simulink model "DYC_controller"  (R2018b)
settings: Solver=FixedStepAuto  StartTime=0.0  StopTime=inf  FixedStep=Ts  RelTol=1e-3  EnableMultiTasking=on
values from neighbouring files (symbols this model uses):
  A_vte = [1 0 -2*Ts*m_s/WB*(l_r*h_rc_f/w1+l_f*h_rc_r/w2) 0 -2*Ts*(K_f/w1+K_r/w2) ... (first row only)    [main.m]
  A_vte_p2 = [1 0 0 0 0 -Ts * m * hc / 2 / WB 0 -Ts * l_r * m * hc / WB / w1 ... (first row only)    [main.m]
  b1 = ones(4,1)/R    [main.m]
  boundary = 3000    [main.m]
  C_vte = [0 1 0 g 0 ... (first row only)    [main.m]
  C_vte_p2 = [1, -1, 1, -1, 0, 0, 0, 0 ... (first row only)    [main.m]
  eta = 0    [main.m]
  F_z1_s = l_r * m * g / 2 / WB    (= 9.45353456158)    [main.m]
  F_z2_s = F_z1_s    (= 9.45353456158)    [main.m]
  F_z3_s = l_f * m * g / 2 / WB    (= 9.11094809852)    [main.m]
  F_z4_s = F_z3_s    (= 9.11094809852)    [main.m]
  g = 9.81    [main.m]
  h_rc_f = 0.00    (= 0)    [main.m]
  h_rc_r = 0.00    (= 0)    [main.m]
  hc = 0.0751    [main.m]
  J = 0.9    [main.m]
  k1 = 2000    [main.m]
  k2 = 1000    [main.m]
  K_f = K_lin*l_cs^2*cos(phi*pi/180)    [main.m]
  K_r = K_lin*l_cs^2*cos(phi*pi/180)    [main.m]
  Kd = 0    [main.m]
  Ki = 75    [main.m]
  Kp = 600    [main.m]
  l_f = 0.1968    [main.m]
  l_r = 0.2042    [main.m]
  m = 3.832    [main.m]
  m_s = 0.9*m    (= 3.4488)    [main.m]
  mu = 0.8    [main.m]
  Protean_PD18_motormap = [2.92104016907 601.978033502 650.789692516 685.109940533 725.756581133 754.659963437 780.850883334 807.9513301 837.761936672 868.484372712 893.788791739 922.70944354 ... (50 elements, 25x2)]    [Protean_PD18_motormap.mat]
  Q_lat_process = 1E0*[var_r^2  0 0 0 0 0 0 0 0 ... (first row only)    [main.m]
  Q_lat_sensor = 1E-2*[var_r_s^2 0 0 0 ... (first row only)    [main.m]
  Q_meas_susp_p1 = [var_ay_m_p^2 0 0 0 ... (first row only)    [main.m]
  Q_meas_susp_p2 = [var_del_Fz^2 0 0 0 0 ... (first row only)    [main.m]
  R = 0.055    [main.m]
  Ts = 0.015    [main.m]
  V_x0 = (1000/3600)*V_x0    (= 11.1111111111)    [main.m]
  w1 = 0.2824    [main.m]
  w2 = 2.929    [main.m]
  WB = 0.406    [main.m]
undefined symbols (not defined in the file or in its folder): C_lf, C_lr, DiscIntNeverNeededParam, Discrete, t_e, Time
libraries: raspberrypilib x24, hdlsllib x21, simulink x17, discretizing x2, ctrlSharedLib x2, sharedTrackingLibrary x1
(part 3 of 3)

== system DYC_controller/Hardware/SSIV Hardware Communication/gyr_z read message (Master --> Slave) ==
  Inport : Inport
  Mux : Mux
      settings: DisplayOption=signals
  Read Bit Set : simulink/Logic and Bit Operations/Bit Set  iBit=7
      settings: SourceProductName=Simulink  SourceProductBaseCode=SL
  uint8_t 1 : Constant  OutDataTypeStr=uint8
  uint8_t 2 : Constant  OutDataTypeStr=uint8
  uint8_t 3 : Constant  OutDataTypeStr=uint8
  Out1 : Outport
  wires:
  uint8_t 2/1 -> Mux/3  "Byte 0 will be returned here"
  Mux/1 -> Out1/1
  uint8_t 3/1 -> Mux/4  "Byte 1 will be returned here"
  Inport/1 -> Read Bit Set/1
  uint8_t 1/1 -> Mux/2  "Junk will be returned here"
  Read Bit Set/1 -> Mux/1  "Addres/RW Byte gyr_z Teensy Status will be returned here"

== system DYC_controller/Hardware/SSIV Hardware Communication/gyr_z return message (Slave --> Master) ==
  In1 : Inport
  8 bytes concatinated converted to double : DataTypeConversion  OutDataTypeStr=double
  Bit Concat : hdlsllib/Logic and Bit Operations/Bit Concat  numInputs=2
      settings: SourceProductName=HDL Coder  SourceProductBaseCode=HD
  Bytes of the return message : Display
      settings: Format=decimal (Stored Integer)
  Data Type Conversion : DataTypeConversion  OutDataTypeStr=int16  RndMeth=Nearest
  Demux : Demux
  Display : Display
      settings: Format=binary (Stored Integer)
  Display1 : Display
      settings: Format=decimal (Stored Integer)
  Display2 : Display
      settings: Format=binary (Stored Integer)
  Gyroscope Int to Double Scale Factor : Gain  Gain=1/900
  gyr_z : Outport
  wires:
  Gyroscope Int to Double Scale Factor/1 -> gyr_z/1, Display1/1
  Demux/3 -> Bit Concat/2
  Demux/4 -> Bit Concat/1
  Bit Concat/1 -> Data Type Conversion/1
  In1/1 -> Demux/1, Bytes of the return message/1
  Demux/1 -> Display/1  "Previous Data"
  Demux/2 -> Display2/1  "Slave Status"
  8 bytes concatinated converted to double/1 -> Gyroscope Int to Double Scale Factor/1  "gyr_z"
  Data Type Conversion/1 -> 8 bytes concatinated converted to double/1

== system DYC_controller/Hardware/SSIV Hardware Communication/radio_steering read message (Master --> Slave) ==
  Inport : Inport
  Mux : Mux
      settings: DisplayOption=signals
  Read Bit Set : simulink/Logic and Bit Operations/Bit Set  iBit=7
      settings: SourceProductName=Simulink  SourceProductBaseCode=SL
  uint8_t 1 : Constant  OutDataTypeStr=uint8
  uint8_t 2 : Constant  OutDataTypeStr=uint8
  uint8_t 3 : Constant  OutDataTypeStr=uint8
  Out1 : Outport
  wires:
  Read Bit Set/1 -> Mux/1  "Addres/RW Byte radio_steering Teensy Status will be returned here"
  uint8_t 1/1 -> Mux/2  "Junk will be returned here"
  Inport/1 -> Read Bit Set/1
  uint8_t 3/1 -> Mux/4  "Byte 1 will be returned here"
  Mux/1 -> Out1/1
  uint8_t 2/1 -> Mux/3  "Byte 0 will be returned here"

== system DYC_controller/Hardware/SSIV Hardware Communication/radio_steering return message (Slave --> Master) ==
  In1 : Inport
  8 bytes concatinated converted to double : DataTypeConversion  OutDataTypeStr=double  RndMeth=Nearest
  Bit Concat : hdlsllib/Logic and Bit Operations/Bit Concat  numInputs=2
      settings: SourceProductName=HDL Coder  SourceProductBaseCode=HD
  Bytes of the return message : Display
      settings: Format=decimal (Stored Integer)
  Data Type Conversion : DataTypeConversion  OutDataTypeStr=int16  RndMeth=Nearest
  Demux : Demux
  Display : Display
      settings: Format=binary (Stored Integer)
  Display1 : Display
      settings: Format=decimal (Stored Integer)
  Display2 : Display
      settings: Format=binary (Stored Integer)
  radio_steering : Outport
  wires:
  8 bytes concatinated converted to double/1 -> Display1/1, radio_steering/1  "radio_steering"
  Demux/2 -> Display2/1  "Slave Status"
  Demux/1 -> Display/1  "Previous Data"
  In1/1 -> Bytes of the return message/1, Demux/1
  Bit Concat/1 -> Data Type Conversion/1
  Demux/4 -> Bit Concat/1
  Demux/3 -> Bit Concat/2
  Data Type Conversion/1 -> 8 bytes concatinated converted to double/1

== system DYC_controller/Hardware/SSIV Hardware Communication/radio_throttle read message (Master --> Slave) ==
  Inport : Inport
  Mux : Mux
      settings: DisplayOption=signals
  Read Bit Set : simulink/Logic and Bit Operations/Bit Set  iBit=7
      settings: SourceProductName=Simulink  SourceProductBaseCode=SL
  uint8_t 1 : Constant  OutDataTypeStr=uint8
  uint8_t 2 : Constant  OutDataTypeStr=uint8
  uint8_t 3 : Constant  OutDataTypeStr=uint8
  Out1 : Outport
  wires:
  Read Bit Set/1 -> Mux/1  "Address/RW Byte radio_throttle Teensy Status will be returned here"
  uint8_t 1/1 -> Mux/2  "Junk will be returned here"
  Inport/1 -> Read Bit Set/1
  uint8_t 3/1 -> Mux/4  "Byte 1 will be returned here"
  Mux/1 -> Out1/1
  uint8_t 2/1 -> Mux/3  "Byte 0 will be returned here"

== system DYC_controller/Hardware/SSIV Hardware Communication/radio_throttle return message (Slave --> Master) ==
  In1 : Inport
  8 bytes concatinated converted to double : DataTypeConversion  OutDataTypeStr=double  RndMeth=Nearest
  Bit Concat : hdlsllib/Logic and Bit Operations/Bit Concat  numInputs=2
      settings: SourceProductName=HDL Coder  SourceProductBaseCode=HD
  Bytes of the return message : Display
      settings: Format=decimal (Stored Integer)
  Data Type Conversion : DataTypeConversion  OutDataTypeStr=int16  RndMeth=Nearest
  Demux : Demux
  Display : Display
      settings: Format=binary (Stored Integer)
  Display1 : Display
      settings: Format=decimal (Stored Integer)
  Display2 : Display
      settings: Format=binary (Stored Integer)
  radio_throttle : Outport
  wires:
  8 bytes concatinated converted to double/1 -> Display1/1, radio_throttle/1  "radio_throttle"
  Demux/2 -> Display2/1  "Slave Status"
  Demux/1 -> Display/1  "Previous Data"
  In1/1 -> Bytes of the return message/1, Demux/1
  Bit Concat/1 -> Data Type Conversion/1
  Demux/4 -> Bit Concat/1
  Demux/3 -> Bit Concat/2
  Data Type Conversion/1 -> 8 bytes concatinated converted to double/1

== system DYC_controller/Hardware/SSIV Hardware Communication/servo_out Write Message (Master --> Slave) ==
  In1 : Inport
  Bit Slice2 : hdlsllib/Logic and Bit Operations/Bit Slice  lidx=15  ridx=8
  Bit Slice3 : hdlsllib/Logic and Bit Operations/Bit Slice  lidx=7  ridx=0
  Display5 : Display
      settings: Format=decimal (Stored Integer)
  Mux : Mux  Inputs=2
      settings: DisplayOption=signals
  Out1 : Outport
  wires:
  In1/1 -> Display5/1, Bit Slice3/1, Bit Slice2/1  "Servo"
  Mux/1 -> Out1/1
  Bit Slice3/1 -> Mux/1
  Bit Slice2/1 -> Mux/2

== system DYC_controller/Hardware/SSIV Hardware Communication/throttle_left_front Write Message (Master --> Slave) ==
  In1 : Inport
  Bit Slice : hdlsllib/Logic and Bit Operations/Bit Slice  lidx=15  ridx=8
  Bit Slice1 : hdlsllib/Logic and Bit Operations/Bit Slice  lidx=7  ridx=0
  Display4 : Display
  Mux : Mux  Inputs=2
      settings: DisplayOption=signals
  Output : Outport
  wires:
  Mux/1 -> Output/1
  Bit Slice/1 -> Display4/1, Mux/2
  Bit Slice1/1 -> Mux/1
  In1/1 -> Bit Slice/1, Bit Slice1/1

== system DYC_controller/Hardware/SSIV Hardware Communication/throttle_left_rear Write Message (Master --> Slave) ==
  In1 : Inport
  Bit Slice : hdlsllib/Logic and Bit Operations/Bit Slice  lidx=15  ridx=8
  Bit Slice1 : hdlsllib/Logic and Bit Operations/Bit Slice  lidx=7  ridx=0
  Display4 : Display
  Mux : Mux  Inputs=2
      settings: DisplayOption=signals
  Output : Outport
  wires:
  In1/1 -> Bit Slice1/1, Bit Slice/1
  Bit Slice1/1 -> Mux/1
  Bit Slice/1 -> Mux/2, Display4/1
  Mux/1 -> Output/1

== system DYC_controller/Hardware/SSIV Hardware Communication/throttle_right_front Write Message (Master --> Slave) ==
  In1 : Inport
  Bit Slice : hdlsllib/Logic and Bit Operations/Bit Slice  lidx=15  ridx=8
  Bit Slice1 : hdlsllib/Logic and Bit Operations/Bit Slice  lidx=7  ridx=0
  Display4 : Display
  Mux : Mux  Inputs=2
      settings: DisplayOption=signals
  Output : Outport
  wires:
  Mux/1 -> Output/1
  Bit Slice/1 -> Display4/1, Mux/2
  Bit Slice1/1 -> Mux/1
  In1/1 -> Bit Slice/1, Bit Slice1/1

== system DYC_controller/Hardware/SSIV Hardware Communication/throttle_right_rear Write Message (Master --> Slave) ==
  In1 : Inport
  Bit Slice : hdlsllib/Logic and Bit Operations/Bit Slice  lidx=15  ridx=8
  Bit Slice1 : hdlsllib/Logic and Bit Operations/Bit Slice  lidx=7  ridx=0
  Display4 : Display
  Mux : Mux  Inputs=2
      settings: DisplayOption=signals
  Output : Outport
  wires:
  In1/1 -> Bit Slice1/1, Bit Slice/1
  Bit Slice1/1 -> Mux/1
  Bit Slice/1 -> Mux/2, Display4/1
  Mux/1 -> Output/1

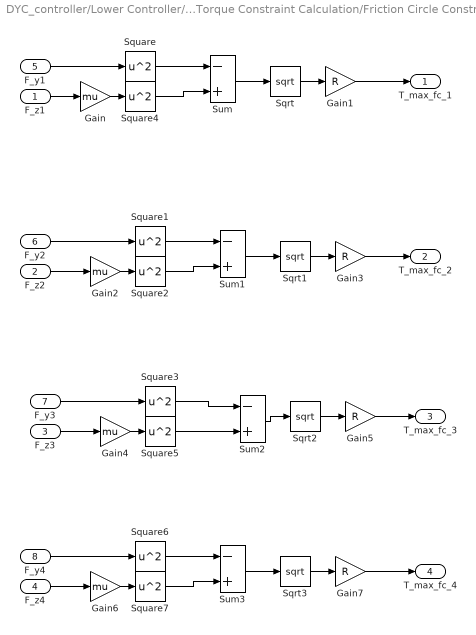
== system DYC_controller/Lower Controller/Torque Constraint Calculation/Friction Circle Constraint ==
  F_z1 : Inport
  F_z2 : Inport  Port=2
  F_z3 : Inport  Port=3
  F_z4 : Inport  Port=4
  F_y1 : Inport  Port=5
  F_y2 : Inport  Port=6
  F_y3 : Inport  Port=7
  F_y4 : Inport  Port=8
  Gain{,2,4,6} (4 alike) : Gain  Gain=mu
  Gain{1,3,5,7} (4 alike) : Gain  Gain=R
  Sqrt{,1..3} (4 alike) : Sqrt  SaturateOnIntegerOverflow=on
  Square{,1..7} (8 alike) : Math  Operator=square  SaturateOnIntegerOverflow=on
  Sum{,1..3} (4 alike) : Sum  Inputs=-+
  T_max_fc_1 : Outport
  T_max_fc_2 : Outport  Port=2
  T_max_fc_3 : Outport  Port=3
  T_max_fc_4 : Outport  Port=4
  wires:
  F_z1/1 -> Gain/1
  Gain3/1 -> T_max_fc_2/1
  F_y1/1 -> Square/1
  Gain/1 -> Square4/1
  Square/1 -> Sum/1
  Square4/1 -> Sum/2
  Sum/1 -> Sqrt/1
  Sqrt/1 -> Gain1/1
  Gain1/1 -> T_max_fc_1/1
  Sqrt1/1 -> Gain3/1
  Sum1/1 -> Sqrt1/1
  Square1/1 -> Sum1/1
  Gain2/1 -> Square2/1
  F_y2/1 -> Square1/1
  F_z2/1 -> Gain2/1
  Square2/1 -> Sum1/2
  Square5/1 -> Sum2/2
  F_z3/1 -> Gain4/1
  F_y3/1 -> Square3/1
  Gain4/1 -> Square5/1
  Square3/1 -> Sum2/1
  Sum2/1 -> Sqrt2/1
  Sqrt2/1 -> Gain5/1
  Gain5/1 -> T_max_fc_3/1
  Gain7/1 -> T_max_fc_4/1
  Sqrt3/1 -> Gain7/1
  Sum3/1 -> Sqrt3/1
  Square6/1 -> Sum3/1
  Gain6/1 -> Square7/1
  F_y4/1 -> Square6/1
  F_z4/1 -> Gain6/1
  Square7/1 -> Sum3/2

== system DYC_controller/Lower Controller/Torque Constraint Calculation/Motor Output Constraint ==
  omega_1 : Inport
  omega_2 : Inport  Port=2
  omega_3 : Inport  Port=3
  omega_4 : Inport  Port=4
  Gain{3..4,11..12} (4 alike) : Gain  Gain=60/(2*pi)
  PD18 Peak Torque : Lookup_n-D  NumberOfTableDimensions=1  BreakpointsForDimension1=Protean_PD18_motormap(:,1)  BreakpointsForDimension3=[5, 7]  Table=Protean_PD18_motormap(:,2)  InternalRulePriority=Speed  RndMeth=Simplest  InputSameDT=on
  n-D Lookup Table1 : Lookup_n-D  NumberOfTableDimensions=1  BreakpointsForDimension1=Protean_PD18_motormap(:,1)  BreakpointsForDimension3=[5, 7]  Table=Protean_PD18_motormap(:,2)  InternalRulePriority=Speed  RndMeth=Simplest  InputSameDT=on
  n-D Lookup Table2 : Lookup_n-D  NumberOfTableDimensions=1  BreakpointsForDimension1=Protean_PD18_motormap(:,1)  BreakpointsForDimension3=[5, 7]  Table=Protean_PD18_motormap(:,2)  InternalRulePriority=Speed  RndMeth=Simplest  InputSameDT=on
  n-D Lookup Table3 : Lookup_n-D  NumberOfTableDimensions=1  BreakpointsForDimension1=Protean_PD18_motormap(:,1)  BreakpointsForDimension3=[5, 7]  Table=Protean_PD18_motormap(:,2)  InternalRulePriority=Speed  RndMeth=Simplest  InputSameDT=on
  T_peak_motor_1 : Outport
  T_peak_motor_2 : Outport  Port=2
  T_peak_motor_3 : Outport  Port=3
  T_peak_motor_4 : Outport  Port=4
  wires:
  Gain3/1 -> PD18 Peak Torque/1
  omega_2/1 -> Gain4/1
  omega_1/1 -> Gain3/1
  Gain4/1 -> n-D Lookup Table1/1
  omega_4/1 -> Gain12/1
  Gain11/1 -> n-D Lookup Table2/1
  Gain12/1 -> n-D Lookup Table3/1
  omega_3/1 -> Gain11/1
  PD18 Peak Torque/1 -> T_peak_motor_1/1
  n-D Lookup Table1/1 -> T_peak_motor_2/1
  n-D Lookup Table2/1 -> T_peak_motor_3/1
  n-D Lookup Table3/1 -> T_peak_motor_4/1

== system DYC_controller/Lower Controller/Torque Constraint Calculation/Road Adhesion Constraint ==
  F_z1 : Inport
  F_z2 : Inport  Port=2
  F_z3 : Inport  Port=3
  F_z4 : Inport  Port=4
  Constant2 : Constant  Value=mu
  Gain6 : Gain  Gain=R
  Multiply{,1..3} (4 alike) : Product
  T_max_ad_1 : Outport
  T_max_ad_2 : Outport  Port=2
  T_max_ad_3 : Outport  Port=3
  T_max_ad_4 : Outport  Port=4
  wires:
  F_z1/1 -> Multiply/2
  F_z2/1 -> Multiply1/2
  F_z3/1 -> Multiply2/2
  Constant2/1 -> Gain6/1
  F_z4/1 -> Multiply3/2
  Gain6/1 -> Multiply/1, Multiply3/1, Multiply2/1, Multiply1/1
  Multiply/1 -> T_max_ad_1/1
  Multiply1/1 -> T_max_ad_2/1
  Multiply2/1 -> T_max_ad_3/1
  Multiply3/1 -> T_max_ad_4/1

== matlab function DYC_controller/Lower Controller/MATLAB Function ==
  settings: updateMethod=DISCRETE
  data: T_max input size=4; torque output size=4; M_des input; T_base input; V_wx input; b1 input; b2 input; C_lf input; C_lr input; R input; fval output; iter output; c_residual output; F_y input; F_z input
function [torque, fval, iter, c_residual] = Torque_Allocation(T_max, M_des, T_base, V_wx, b1, b2, C_lf, C_lr, R, F_y, F_z)
% This function solves a constrained optimization problem for optimal
% torque allocation which satisfies the yaw moment control signal
% Cost function: longitudinal slip power loss
% Method: Lagrangian algorithm
% Reference: Wei-Ta Chu, "Algorithms for Constrained Optimization"

V_wx_1 = V_wx(1);
V_wx_2 = V_wx(2);
V_wx_3 = V_wx(3);
V_wx_4 = V_wx(4);

C_l1 = C_lf;
C_l2 = C_lf;
C_l3 = C_lr;
C_l4 = C_lr;

T_min = - T_max;
x      = [0 0 0 0]';    % Initial guess for torque values

% Concatenate torque vectoring model vectors
B_TV = [ b1, b2 ]';
A    = B_TV;                    % Coefficient matrix
c    = [ T_base / R, M_des ]';       % Vector of control objectives
D    = [ V_wx_1 / (R ^ 2 * C_l1), 0, 0, 0;  % Slip power loss matrix
         0, V_wx_2 / (R ^ 2 * C_l2), 0, 0;
         0, 0, V_wx_3 / (R ^ 2 * C_l3), 0;
         0, 0, 0, V_wx_4 / (R ^ 2 * C_l4) ];

% T    = @(x) [x(1) x(2) x(3) x(4)]';
% Y    = @(F_y) [F_y(1) F_y(2) F_y(3) F_y(4)]';
% Z    = @(F_z) [1/F_z(1) 1/F_z(2) 1/F_z(3) 1/F_z(4)];
% X    = @(x) [x(1) 0 0 0;
%              0 x(2) 0 0;
%              0 0 x(3) 0;
%              0 0 0 x(4)];
% W    = @(F_y) [F_y(1) 0 0 0;
%                0 F_y(2) 0 0;
%                0 0 F_y(3) 0;
%                0 0 0 F_y(4)];
%      
  
% Objective function F(x) to minimize
% Slip power loss
F  = @(x) x' * D * x;
dF = @(x) 2 * D * x;

% % Vertical load matching
% F = @(x, F_z) 0.5*x'*Q*x + (x(1)/(x(1)+x(3)) - (F_z(1)/(F_z(1) + F_z(3))))^2 + (x(2)/(x(2)+x(4))...
%     -F_z(2)/(F_z(2)+F_z(4)))^2;
% 
% dF = @(x, F_z) [-2*(x(1)/(x(1) + x(3)) - F_z(1)/(F_z(1) + F_z(3)))*(x(1)/(x(1) + x(3))^2 -...
%                 1/(x(1) + x(3)));
%                 -2*(x(2)/(x(2) + x(4)) - F_z(2)/(F_z(2) + F_z(4)))*(x(2)/(x(2) + x(4))^2 -...
%                 1/(x(2) + x(4)));
%                 -(2*x(1)*(x(1)/(x(1) + x(3)) - F_z(1)/(F_z(1) + F_z(3))))/(x(1) + x(3))^2;
%                 -(2*x(2)*(x(2)/(x(2) + x(4)) - F_z(2)/(F_z(2) + F_z(4))))/(x(2) + x(4))^2];

% % Total force coefficient
% F = @(x, F_y, F_z) Z(F_z) * (X(x) * T(x) / R .^ 2 + W(F_y) * Y(F_y)) .^ 0.5;
% 
% % Gradient of F
% dF = @(x, F_y, F_z) [x(1)/(F_z(1)*R^2*(F_y(1)^2 + x(1)^2/R^2)^(1/2));
%                      x(2)/(F_z(2)*R^2*(F_y(2)^2 + x(2)^2/R^2)^(1/2));
%                      x(3)/(F_z(3)*R^2*(F_y(3)^2 + x(3)^2/R^2)^(1/2));
%                      x(4)/(F_z(4)*R^2*(F_y(4)^2 + x(4)^2/R^2)^(1/2))];

% Constrained gradient descent parameters
alpha    = .50;     % Learning rate for torque updates
kappa    = .01;     % Learning rate for equality Lagrange multiplier updates1
gamma    = .01;      % Learning rate for inequality Lagrange multiplier updates
max_iter = 50000;   % Set the maximum number of iterations before exiting
func_tol = 1E-5;     % Termination tolerance for F(x)

fvals       = zeros(max_iter, 1); % store F(x) values across iterations

% Iterate
lambda      = [ 0, 0 ]';            % Initial guess for equality Lagrange multipliers
mu_1        = [0, 0, 0, 0]';        % Initial guess for inequality Lagrange multiplier #1 update
mu_2        = [0, 0, 0, 0]';        % Initial guess for inequality Lagrange multiplier #2 update
iter        = 1;                    % Iterations counter
% fvals       = [];
step        = [10 10 10 10]';                   % Initialize step larger than func_tol
fvals(iter) = F(x);

while iter < max_iter && any(abs(step) > func_tol)
    iter   = iter + 1;
    current_x = x;
    % Update Lagrange multipliers
    lambda      = lambda + kappa * (A * current_x - c);
    mu_1        = max(mu_1 + gamma * (T_min - current_x), [0, 0, 0, 0]');
    mu_2        = max(mu_2 + gamma * (current_x - T_max), [0, 0, 0, 0]');
    fvals(iter) = F(current_x);  % Evaluate objective function
    x    = current_x + alpha * (-dF(current_x) - A' * lambda + mu_1 - mu_2);  % Gradient descent
    step      = x - current_x;
end

c_residual = A * x - c;
fval = fvals(iter); 
torque = x;

== matlab function DYC_controller/Force Estimator/Vertical Tire Force Estimation/MATLAB Function ==
  data: x input; f output
function f = vertical_force_nonlin_model(x)
% Nonlinear function describing the lateral weight transfer of a vehicle

% Vehicle Parameters
m  = 1400; % Vehicle mass [kg]

% Vehicle geometry
WB  = 2.88;     % Wheelbase [m]
l_f = 1.1907;   % Distance from CG to front axle
l_r = WB-l_f;   % Distance from CG to rear axle
w1 = 1.565;     % Front track width [m]
w2 = 1.565;     % Rear track width [m]
h_c = 0.60;       % Height of the CG
t_e = 0.05;     % sampling time
g   = 9.81;

x1 = x(1);  % F_z1
x2 = x(2);  % F_z2
x3 = x(3);  % F_z3
x4 = x(4);  % F_z4
x5 = x(5);  % a_x
x6 = x(6);  % a_x_dot
x7 = x(7);  % a_y
x8 = x(8);  % a_y_dot

f = [x1+t_e*(-h_c*m/2/WB*x6-m*l_r*h_c/WB/w1*x8+m*h_c^2/WB/w1/g*x5*x8+m*h_c^2/WB/w1/g*x6*x7);
     x2+t_e*(-h_c*m/2/WB*x6+m*l_r*h_c/WB/w1*x8-m*h_c^2/WB/w1/g*x5*x8-m*h_c^2/WB/w1/g*x6*x7);
     x3+t_e*(h_c*m/2/WB*x6-m*l_r*h_c/WB/w2*x8-m*h_c^2/WB/w2/g*x5*x8-m*h_c^2/WB/w2/g*x6*x7);
     x4+t_e*(h_c*m/2/WB*x6+m*l_r*h_c/WB/w2*x8+m*h_c^2/WB/w2/g*x5*x8+m*h_c^2/WB/w2/g*x6*x7);
     x5+t_e*x6;
     x6;
     x7+t_e*x8;
     x8];


end

== matlab function DYC_controller/Force Estimator/Vertical Tire Force Estimation/MATLAB Function1 ==
  data: x input; j output
function j = vertical_force_jacobian(x)
%UNTITLED3 Summary of this function goes here
%   Detailed explanation goes here

% Vehicle Parameters
m  = 1400; % Vehicle mass [kg]

% Vehicle geometry
WB  = 2.88;     % Wheelbase [m]
l_f = 1.1907;   % Distance from CG to front axle
l_r = WB-l_f;   % Distance from CG to rear axle
w1 = 1.565;     % Front track width [m]
w2 = 1.565;     % Rear track width [m]
h_c = 0.60;       % Height of the CG
t_e = 0.05;     % sampling rate
g   = 9.81;

x6 = x(6);  % a_x_dot
x7 = x(7);  % a_y
x8 = x(8);  % a_y_dot

j  = [1 0 0 0 0 0 0 0;
      0 1 0 0 0 0 0 0;
      0 0 1 0 0 0 0 0;
      0 0 0 1 0 0 0 0;
      m*h_c^2/WB/w1/g*x8 -t_e*m*h_c^2/WB/w1/g*x8 -t_e*m*h_c^2/WB/w2/g*x8 t_e*m*h_c^2/WB/w2/g*x8 1 0 0 0;
      t_e*(m*(-h_c/2/WB+h_c^2/WB/w1/g*x7)) t_e*(m*(-h_c/2/WB-h_c^2/WB/w1/g*x7)) t_e*(m*(h_c/2/WB-h_c^2/WB/w2/g*x7)) t_e*(m*(h_c/2/WB+h_c^2/WB/w2/g*x7)) t_e 1 0 0;
      t_e*m*h_c^2/WB/w1/g*x6 -t_e*m*h_c^2/WB/w1/g*x6 -t_e*m*h_c^2/WB/w2/g*x6 t_e*m*h_c^2/WB/w2/g*x6 0 0 1 0;
      -m*l_r*h_c/WB/w1 m*l_r*h_c/WB/w1 -m*l_f*h_c/WB/w2 m*l_f*h_c/WB/w2 0 0 t_e 1];
  
end

== matlab function DYC_controller/Force Estimator/Vertical Tire Force Estimation/MATLAB Function2 ==
  data: x input; h output
function h = vertical_force_nonlin_measurement_model(x)
%UNTITLED2 Summary of this function goes here
%   Detailed explanation goes here
x1 = x(1);  % F_z1
x2 = x(2);  % F_z2
x3 = x(3);  % F_z3
x4 = x(4);  % F_z4
x5 = x(5);  % a_x
x6 = x(6);  % a_x_dot
x7 = x(7);  % a_y
x8 = x(8);  % a_y_dot

h = [x1 - x2 + x3 - x4;
     x1 + x2;
     x5;
     x7;
     x1 + x2 + x3 + x4];

end

== matlab function DYC_controller/Force Estimator/Lateral Tire Force Estimation/MATLAB Function ==
  data: X_E input; U input; X_P output; P_P output; Z_P output; Kk output; Pz_P output; P_E input; Q_lat_process input; Q_lat_sensor input
function [X_P, P_P, Z_P, Kk, Pz_P] = lateral_prediction_UKF(X_E, U, P_E, Q_lat_process, Q_lat_sensor)

% Vehicle Parameters
m  = 1400; % Vehicle mass [kg]
Iz = 2000;   % Yaw inertia

% Vehicle geometry
WB  = 2.88;     % Wheelbase [m]
l_f = 1.1907;   % Distance from CG to front axle
l_r = WB-l_f;   % Distance from CG to rear axle
w1 = 1.565;     % Front track width [m]
w2 = 1.565;     % Rear track width [m]
mu = 0.8;       % Friction coefficient
t_e_lat = .005;     % Kalman sampling rate

% Tire Stiffness
C_af = 40000 ;    % Front cornering stiffness [N/rad]
C_ar = 35000;    % Rear cornering stiffness [N/rad]
sigma_1 = 0.5;   % Front relaxation length [m]
sigma_2 = 0.5;   % Rear relaxation length [m]

% Model
ALF = @(X, U) [U(1) - atan((X(3,:) + l_f .* X(1,:)) ./ (X(2,:)-w1/2.*X(1,:)));
               U(1) - atan((X(3,:) + l_f .* X(1,:)) ./ (X(2,:)+w1/2.*X(1,:)));
                    - atan((X(3,:) - l_r .* X(1,:)) ./ (X(2,:)-w2/2.*X(1,:)));
                    - atan((X(3,:) - l_r .* X(1,:)) ./ (X(2,:)+w2/2.*X(1,:)))];

LAM = @(ALF, U) [mu .* U(2) / 2 / C_af ./ abs(tan(ALF(1,:)));
                 mu .* U(3) / 2 / C_af ./ abs(tan(ALF(2,:)));
                 mu .* U(4) / 2 / C_ar ./ abs(tan(ALF(3,:)));
                 mu .* U(5) / 2 / C_ar ./ abs(tan(ALF(4,:)))];
            
F_y_bar = @(ALF, f_LAM) [C_af .* tan(ALF(1,:)) .* f_LAM(1,:);
                         C_af .* tan(ALF(2,:)) .* f_LAM(2,:);
                         C_ar .* tan(ALF(2,:)) .* f_LAM(3,:);
                         C_ar .* tan(ALF(2,:)) .* f_LAM(4,:)];
                      
f = @(X, U, F_y_bar) [X(1,:) + t_e_lat ./ Iz .* (l_f * (X(4,:) + X(5,:)) .* cos(U(1))...
     + X(8,:) .* sin(U(1)) - l_r .* (X(6,:) + X(7,:)) + w2 ./ 2 .*...
     ((X(4,:)- X(5,:)) .* sin(U(1)) + X(8,:) .* U(3) / (U(2) + U(3)) .* cos(U(1))...
     -X(8,:) .* U(2) / (U(2) + U(3)) * cos(U(1)) + X(9,:) .* U(5) / (U(4) + U(5))...
     -X(9,:) .* U(4) / (U(4) + U(5))));
     
     X(2,:) + t_e_lat / m .* (X(8,:) .* cos(U(1)) -...
     (X(4,:) + X(5,:)) .* sin(U(1)) + X(9,:))+ t_e_lat .* X(1,:) .* X(3,:);
     
     X(3,:) + t_e_lat / m .* (X(8,:) .* sin(U(1)) + (X(4,:) + X(5,:)) .* cos(U(1)) +...
     X(6,:) + X(7,:)) - t_e_lat .* X(1,:) .* X(2,:);
     
     X(4,:) + t_e_lat .* X(2,:) / sigma_1 .* (X(4,:) + F_y_bar(1,:));
     
     X(5,:) + t_e_lat .* X(2,:) / sigma_1 .* (X(5,:) + F_y_bar(2,:));
     
     X(6,:) + t_e_lat .* X(2,:) / sigma_2 .* (X(6,:) + F_y_bar(3,:));
     
     X(7,:) + t_e_lat .* X(2,:) / sigma_2 .* (X(7,:) + F_y_bar(4,:));
     
     X(8,:);
     
     X(9,:)];

h = @(X,U) [X(1,:);
            X(2,:);
            1 / m .* (-(X(4,:) + X(5,:)) .* sin(U(1)) + X(8,:) * cos(U(1))...
            + X(9,:));
            1 / m .* ((X(4,:) + X(5,:)) .* cos(U(1)) + X(6,:) + X(7,:) + ...
            X(8,:) * sin(U(1)))];
 
% UKF Parameters
L=length(X_E);
chi_E = zeros(L,2*L+1);
W_m   = zeros(1,2*L+1);
W_c   = zeros(1,2*L+1);

%Scaling parameters to generate sigma points
alpha=1;
k=0;
beta=2;

lambda=alpha^2*(L+k)-L;

% Matrix definition
f_lt = zeros(4,2*L+1);

% Sigma Points and corresponding weights
chi_E(:,1)=X_E;
W_m(1)=lambda/(L+lambda);
W_c(1)=lambda/(L+lambda)+(1-alpha^2+beta);
A = chol(P_E);

for ii=1:L
    temp=((L+lambda))^0.5*A;
    chi_E(:,ii+1)=X_E+temp(ii,:)';
    W_m(ii+1)=1/(2*(L+lambda));
    W_c(ii+1)=1/(2*(L+lambda));
end

for ii=L+1:2*L
    temp=((L+lambda))^0.5*A;
    chi_E(:,ii+1)=X_E-temp(ii-L,:)';
    W_m(ii+1)=1/(2*(L+lambda));
    W_c(ii+1)=1/(2*(L+lambda));
end
    
% Predict state for each sigma point
slip = ALF(chi_E, U);
lambda_tire = LAM(slip, U);
for i = 1:4
    for j = 1:(2*L+1)
        if lambda_tire(i,j) < 1
            f_lt(i,j) = (2-lambda_tire(i,j))*lambda_tire(i,j);
        else
            f_lt(i,j) = 1;
        end
    end
end
% f_lt = f_LAM(lambda_tire);
F_y_qs = F_y_bar(slip, f_lt);

chi_P=f(chi_E, U, F_y_qs);           
zed_P = h(chi_E, U);

% Compute mean and variance for sigma points 
P_P=Q_lat_process;
X_P=chi_P*W_m';
for ii=1:2*L+1
    P_P=P_P+W_c(ii)*(chi_P(:,ii)-X_P)*(chi_P(:,ii)-X_P)';
end

Pz_P=Q_lat_sensor;
Z_P=zed_P*W_m';
for ii=1:2*L+1
    Pz_P=Pz_P+W_c(ii)*(zed_P(:,ii)-Z_P)*(zed_P(:,ii)-Z_P)';
end

Pxz_P=zeros(9,4);
for ii=1:2*L+1
    Pxz_P=Pxz_P+W_c(ii)*(chi_P(:,ii)-X_P)*(zed_P(:,ii)-Z_P)';
end

% Compute Kalman Gain
Kk=Pxz_P/Pz_P;

== matlab function DYC_controller/Force Estimator/Lateral Tire Force Estimation/MATLAB Function1 ==
  data: Pz_P input; X_E output; Z_P input; X_P input; P_P input; Y input; Kk input; P_E output
% The data is courtesy of the LIVIC laboratory at IFSTTAR in Paris France.
% The m-files have been originally written by Dr Dominique Gruyer at the LIVIC, IFSTTAR
% Adapted by Denis Gingras at the Université de Sherbrooke.


function [X_E,P_E]=lateral_estimation_UKF(Pz_P,Z_P,X_P,P_P,Y,Kk)

% P_P: varcov matrix on prediction
% Hk: measurement equations matrix, selects state variables that are estimated (update)
% X_P: Prediction used
% Y_GPS: GPS data, (X,Y)
% Q_GPS: GPS noise

%==================================
% ESTIMATION STEP: instant k/k
%==================================

% Compute Estimate
X_E=X_P+Kk*(Y-Z_P);

% Compute error covariance
P_E=P_P-Kk*Pz_P*Kk';

end
